simulink model "arduino_simulink_pid"  (R2021a)
settings: Solver=FixedStepAuto  StartTime=0.0  StopTime=10  RelTol=1e-3  EnableMultiTasking=on
libraries: arduinolib x3
settings Model: SILPILModeSetting=veronly  ExtModeTrigDuration=2  Creator=Hp  LastModifiedBy=Hp
settings OptimizationCC: EnhancedBackFolding=on  PassReuseOutputArgsAs=Individual arguments  ZeroExternalMemoryAtStartup=off  ZeroInternalMemoryAtStartup=off  MaxStackSize=64  OptimizeBlockOrder=speed  DifferentSizesBufferReuse=on  OptimizationCustomize=off  EfficientTunableParamExpr=on
settings DebuggingCC: ParameterTunabilityLossMsg=error
settings HardwareCC: ProdBitPerInt=16  ProdBitPerPointer=16  ProdBitPerSizeT=16  ProdBitPerPtrDiffT=16  ProdLargestAtomicFloat=None  ProdWordSize=8  ProdHWDeviceType=Atmel->AVR
settings SFSimCC: MATLABDynamicMemAlloc=off
settings RTWCC: SystemTargetFile=ert.tlc  HardwareBoard=Arduino Uno  TemplateMakefile=ert_default_tmf  Toolchain=Arduino AVR  BuildConfiguration=Faster Runs
settings CodeAppCC: ForceParamTrailComments=on  IgnoreCustomStorageClasses=off  OperatorAnnotations=on  SimulinkDataObjDesc=on  SFDataObjDesc=on  InsertBlockDesc=on
settings ERTTargetCC: SupportContinuousTime=on  SupportVariableSizeSignals=on  ExtModeStaticAllocSize=250

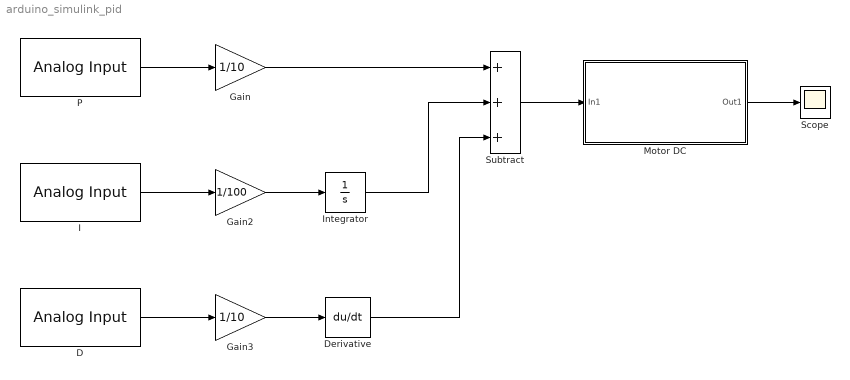
== system arduino_simulink_pid ==
  D : arduinolib/Analog Input  pinNumber=2  ReadResultsOnly=off  ConversionTriggerSource=Software  ExternalTriggerType=uint32( 0 )  OutputDataType=uint16  EnableConversionCompleteNotify=off  EnableOuputStatus=off  SampleTime=0.01  blockPlatform=arduino
  Derivative : Derivative
  Gain : Gain  Gain=1/10  ParamDataTypeStr=double
  Gain2 : Gain  Gain=1/100  ParamDataTypeStr=double
  Gain3 : Gain  Gain=1/10  OutDataTypeStr=double
  I : arduinolib/Analog Input  pinNumber=1  ReadResultsOnly=off  ConversionTriggerSource=Software  ExternalTriggerType=uint32( 0 )  OutputDataType=uint16  EnableConversionCompleteNotify=off  EnableOuputStatus=off  SampleTime=0.01  blockPlatform=arduino
  Integrator : Integrator
  Motor DC : Subsystem
  P : arduinolib/Analog Input  pinNumber=0  ReadResultsOnly=off  ConversionTriggerSource=Software  ExternalTriggerType=uint32( 0 )  OutputDataType=uint16  EnableConversionCompleteNotify=off  EnableOuputStatus=off  SampleTime=0.01  blockPlatform=arduino
  Scope : Scope
  Subtract : Sum  Inputs=+++
  wires:
  P/1 -> Gain/1
  I/1 -> Gain2/1
  D/1 -> Gain3/1
  Gain3/1 -> Derivative/1
  Gain2/1 -> Integrator/1
  Motor DC/1(Out1) -> Scope/1
  Gain/1 -> Subtract/1
  Subtract/1 -> Motor DC/1(In1)
  Integrator/1 -> Subtract/2
  Derivative/1 -> Subtract/3

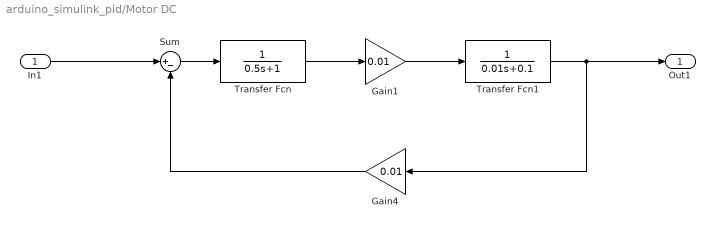
== system arduino_simulink_pid/Motor DC ==
  In1 : Inport
  Gain1 : Gain  Gain=0.01
  Gain4 : Gain  Gain=0.01
  Sum : Sum  Inputs=|+-
  Transfer Fcn : TransferFcn  Denominator=[0.5 1]
  Transfer Fcn1 : TransferFcn  Denominator=[0.01 0.1]
  Out1 : Outport
  wires:
  Gain1/1 -> Transfer Fcn1/1
  Transfer Fcn1/1 -> Out1/1, Gain4/1
  Transfer Fcn/1 -> Gain1/1
  In1/1 -> Sum/1
  Gain4/1 -> Sum/2
  Sum/1 -> Transfer Fcn/1
